simulink model "isubsystem_main"  (R2014b)
settings: Solver=ode45  StartTime=0.0  StopTime=5  FixedStep=0.001  RelTol=1e-3
undefined symbols (not defined in the file): v1, v10, v11, v12, v13, v14, v15, v16, v17, v18, v19, v2, v20, v21, v22, v3, v4, v5, v6, v7, v8, v9
(part 1 of 2)
settings Model: Creator=QiuJiongzhi  LastModifiedBy=QiuJiongzhi
settings SolverCC: ZeroCrossControl=DisableAll

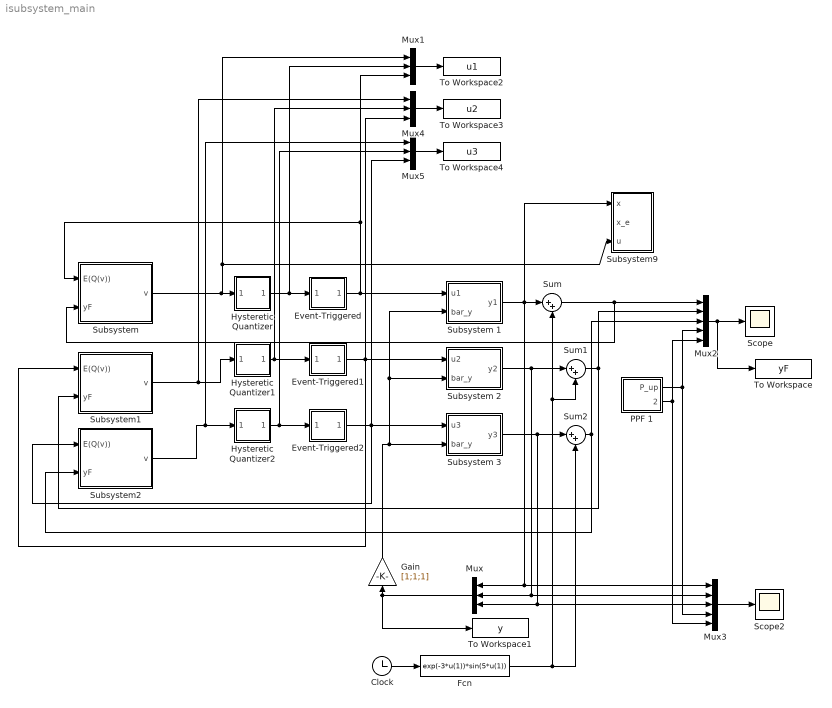
== system isubsystem_main ==
  Clock : Clock
  Event-Triggered : Subsystem
      mask Display: fprintf('E(μ)');
  Event-Triggered1 : Subsystem
      mask Display: fprintf('E(μ)');
  Event-Triggered2 : Subsystem
      mask Display: fprintf('E(μ)');
  Fcn : Fcn  Expr=exp(-3*u(1))*sin(5*u(1))
  Gain : Gain  Gain=[1;1;1]
  Hysteretic Quantizer : Subsystem
      mask Display: fprintf('Q(μ)')
  Hysteretic Quantizer1 : Subsystem
      mask Display: fprintf('Q(μ)')
  Hysteretic Quantizer2 : Subsystem
      mask Display: fprintf('Q(μ)')
  Mux{,1,4..5} (4 alike) : Mux  Inputs=3
  Mux2 : Mux  Inputs=5
  Mux3 : Mux  Inputs=5
  PPF 1 : Subsystem  mask{psi0=1, psiinf=0.05, T=1.5, q=0.1}
  Scope : Scope
      settings: ShowLegends=on  YMin=-1  YMax=1
  Scope2 : Scope
      settings: ShowLegends=on  YMin=-1  YMax=1  SaveName=ScopeData3
  Subsystem : Subsystem
  Subsystem 1 : Subsystem  mask{x1_0=0.5, x2_0=0.3}
      mask prompts: x1_0 "x1(0)"; x2_0 "x2(0)"
  Subsystem 2 : Subsystem  mask{x1_0=0.5, x2_0=0.45}
      mask prompts: x1_0 "x1(0)"; x2_0 "x2(0)"
  Subsystem 3 : Subsystem  mask{x1_0=0.5, x2_0=0.3}
      mask prompts: x1_0 "x1(0)"; x2_0 "x2(0)"
  Subsystem1 : Subsystem
  Subsystem2 : Subsystem
  Subsystem9 : Subsystem
  Sum : Sum  Inputs=|++
  Sum1 : Sum  Inputs=|++
  Sum2 : Sum  Inputs=|++
  To Workspace : ToWorkspace  VariableName=yF  SaveFormat=Structure With Time  SampleTime=-1
  To Workspace1 : ToWorkspace  VariableName=y  SaveFormat=Structure With Time  SampleTime=-1
  To Workspace2 : ToWorkspace  VariableName=u1  SaveFormat=Structure With Time  SampleTime=-1
  To Workspace3 : ToWorkspace  VariableName=u2  SaveFormat=Structure With Time  SampleTime=-1
  To Workspace4 : ToWorkspace  VariableName=u3  SaveFormat=Structure With Time  SampleTime=-1
  wires:
  Sum/1 -> Mux2/1, Subsystem/2(yF)
  Clock/1 -> Fcn/1
  Fcn/1 -> Sum1/2, Sum/2, Sum2/2
  Mux/1 -> To Workspace1/1, Gain/1
  Mux1/1 -> To Workspace2/1
  Hysteretic Quantizer/1(Q(\miu)) -> Mux1/2, Event-Triggered/1(In1)
  Event-Triggered/1(Out1) -> Mux1/3, Subsystem/1(E(Q(v))), Subsystem 1/1(u1)
  Subsystem 2/1(y2) -> Mux/2, Mux3/2, Sum1/1
  Subsystem 3/1(y3) -> Mux3/3, Mux/3, Sum2/1
  Subsystem/1(v) -> Mux1/1, Subsystem9/3(u), Hysteretic Quantizer/1(\miu)
  Event-Triggered1/1(Out1) -> Mux4/3, Subsystem1/1(E(Q(v))), Subsystem 2/1(u2)
  Hysteretic Quantizer1/1(Q(\miu)) -> Event-Triggered1/1(In1), Mux4/2
  Subsystem1/1(v) -> Mux4/1, Hysteretic Quantizer1/1(\miu)
  Sum1/1 -> Subsystem1/2(yF), Mux2/2
  Hysteretic Quantizer2/1(Q(\miu)) -> Mux5/2, Event-Triggered2/1(In1)
  Event-Triggered2/1(Out1) -> Mux5/3, Subsystem2/1(E(Q(v))), Subsystem 3/1(u3)
  Subsystem2/1(v) -> Mux5/1, Hysteretic Quantizer2/1(\miu)
  Sum2/1 -> Subsystem2/2(yF), Mux2/3
  Gain/1 -> Subsystem 3/2(bar_y), Subsystem 2/2(bar_y), Subsystem 1/2(bar_y)
  Mux2/1 -> To Workspace/1, Scope/1
  PPF 1/1(P_up) -> Mux2/4, Mux3/4
  PPF 1/2("P_down ") -> Mux2/5, Mux3/5
  Mux3/1 -> Scope2/1
  Subsystem 1/1(y1) -> Sum/1, Mux3/1, Mux/1, Subsystem9/1(x)
  Mux4/1 -> To Workspace3/1
  Mux5/1 -> To Workspace4/1

== system isubsystem_main/Event-Triggered ==
  In1 : Inport
  MATLAB Function : MATLAB Function  TreatAsAtomicUnit=on
  Mux : Mux  Inputs=2
  Scope : Scope
  To Workspace : ToWorkspace  VariableName=triger1  SaveFormat=Structure With Time  SampleTime=-1
  Unit Delay : UnitDelay  SampleTime=-1
  Out1 : Outport
  wires:
  Unit Delay/1 -> MATLAB Function/2(miu_tk)
  In1/1 -> MATLAB Function/1(miu)
  MATLAB Function/1(E_out) -> Unit Delay/1, Out1/1
  Mux/1 -> Scope/1
  MATLAB Function/2(eta) -> Mux/1
  MATLAB Function/3(triger) -> To Workspace/1, Mux/2

== system isubsystem_main/Event-Triggered1 ==
  In1 : Inport
  MATLAB Function : MATLAB Function  TreatAsAtomicUnit=on
  Mux : Mux  Inputs=2
  Scope : Scope
  To Workspace : ToWorkspace  VariableName=triger2  SaveFormat=Structure With Time  SampleTime=-1
  Unit Delay : UnitDelay  SampleTime=-1
  Out1 : Outport
  wires:
  Unit Delay/1 -> MATLAB Function/2(miu_tk)
  In1/1 -> MATLAB Function/1(miu)
  MATLAB Function/1(E_out) -> Unit Delay/1, Out1/1
  Mux/1 -> Scope/1
  MATLAB Function/2(eta) -> Mux/1
  MATLAB Function/3(triger) -> To Workspace/1, Mux/2

== system isubsystem_main/Event-Triggered2 ==
  In1 : Inport
  MATLAB Function : MATLAB Function  TreatAsAtomicUnit=on
  Mux : Mux  Inputs=2
  Scope : Scope
  To Workspace : ToWorkspace  VariableName=triger3  SaveFormat=Structure With Time  SampleTime=-1
  Unit Delay : UnitDelay  SampleTime=-1
  Out1 : Outport
  wires:
  Unit Delay/1 -> MATLAB Function/2(miu_tk)
  In1/1 -> MATLAB Function/1(miu)
  MATLAB Function/1(E_out) -> Unit Delay/1, Out1/1
  Mux/1 -> Scope/1
  MATLAB Function/2(eta) -> Mux/1
  MATLAB Function/3(triger) -> To Workspace/1, Mux/2

== system isubsystem_main/Hysteretic Quantizer ==
  \miu : Inport
  Derivative : Derivative
  MATLAB Function : MATLAB Function  TreatAsAtomicUnit=on
  Unit Delay : UnitDelay  SampleTime=-1
  Q(\miu) : Outport
  wires:
  Unit Delay/1 -> MATLAB Function/2(Output_t)
  \miu/1 -> Derivative/1, MATLAB Function/1(miu)
  MATLAB Function/1(Q_miu) -> Q(\miu)/1, Unit Delay/1
  Derivative/1 -> MATLAB Function/3(dmiu)

== system isubsystem_main/Hysteretic Quantizer1 ==
  \miu : Inport
  Derivative : Derivative
  MATLAB Function : MATLAB Function  TreatAsAtomicUnit=on
  Unit Delay : UnitDelay  SampleTime=-1
  Q(\miu) : Outport
  wires:
  Unit Delay/1 -> MATLAB Function/2(Output_t)
  \miu/1 -> Derivative/1, MATLAB Function/1(miu)
  MATLAB Function/1(Q_miu) -> Q(\miu)/1, Unit Delay/1
  Derivative/1 -> MATLAB Function/3(dmiu)

== system isubsystem_main/Hysteretic Quantizer2 ==
  \miu : Inport
  Derivative : Derivative
  MATLAB Function : MATLAB Function  TreatAsAtomicUnit=on
  Unit Delay : UnitDelay  SampleTime=-1
  Q(\miu) : Outport
  wires:
  Unit Delay/1 -> MATLAB Function/2(Output_t)
  \miu/1 -> Derivative/1, MATLAB Function/1(miu)
  MATLAB Function/1(Q_miu) -> Q(\miu)/1, Unit Delay/1
  Derivative/1 -> MATLAB Function/3(dmiu)

== system isubsystem_main/PPF 1 ==
  Clock1 : Clock
  Constant : Constant  Value=psi0
  Constant1 : Constant  Value=psiinf
  Constant2 : Constant  Value=q
  Constant3 : Constant  Value=T
  MATLAB Function : MATLAB Function  TreatAsAtomicUnit=on
  Saturation : Saturate  UpperLimit=1  LowerLimit=-1
  Saturation1 : Saturate  UpperLimit=1  LowerLimit=-1
  P_up : Outport
  "P_down " : Outport  Port=2
  wires:
  MATLAB Function/1(P_up) -> Saturation/1
  MATLAB Function/2(P_down) -> Saturation1/1
  Clock1/1 -> MATLAB Function/5(t)
  Constant2/1 -> MATLAB Function/4(q)
  Constant1/1 -> MATLAB Function/2(psiinf)
  Constant/1 -> MATLAB Function/1(psi0)
  Constant3/1 -> MATLAB Function/3(T)
  Saturation/1 -> P_up/1
  Saturation1/1 -> "P_down "/1

== system isubsystem_main/Subsystem ==
  E(Q(v)) : Inport
  yF : Inport  Port=2
  Controller1 : Subsystem  mask{k2=v1, b_low=1, b_high=1, li=1, sigma=v2, gamma1=v3, epsilon10=v4, epsilon11=v5, epsilon12=v6, epsilon13=v7, epsilon14=v8, epsilon15=v9, eta0=v10, gamma2=v11, epsilon20=v12, epsilon22=v13, epsilon23=v14, epsilon24=v15, epsilon25=v16, l1=0.2, l2=1.5, w=v17}
      mask DialogControl Container3 Prompt: α_1
      mask DialogControl Container3_copy Prompt: α_n
      mask DialogControl Container4 Prompt: Q(v)
  Fuzzy : Subsystem  mask{Psi=1, eta1=v22}
  "PPF " : Subsystem  mask{psi0=1, psiinf=0.05, T=1.5, q=0.1}
  reduced-order dynamic gain observer : Subsystem  mask{k2=v1, sigma=v2, theta=v18, K=v19, P=1, lP=1, epsilon1=v20, epsilon2=v21, epsilon10=v4, epsilon20=v12, vartheta=0.05}
  v : Outport
  wires:
  Fuzzy/2(Xi) -> Controller1/8(Xi)
  Fuzzy/1(dW) -> Controller1/7(dW)
  reduced-order dynamic gain observer/2(lambda2) -> Controller1/6(lambda2)
  reduced-order dynamic gain observer/1(dL) -> Controller1/5(dL)
  "PPF "/2("dpsi ") -> Controller1/3(dpsi)
  Controller1/1(v) -> v/1
  "PPF "/1(psi) -> Controller1/2(psi)
  "PPF "/3(ddpsi) -> Controller1/4(ddpsi)
  Controller1/2(z1) -> Fuzzy/2(z1)
  E(Q(v))/1 -> reduced-order dynamic gain observer/1(u)
  yF/1 -> Fuzzy/1(yF), Controller1/1(yF), reduced-order dynamic gain observer/2(yF)

== system isubsystem_main/Subsystem 1 ==
  u1 : Inport
  bar_y : Inport  Port=2
  Integrator : Integrator  InitialCondition=x1_0
  Integrator1 : Integrator  InitialCondition=x2_0
  MATLAB Function : MATLAB Function  TreatAsAtomicUnit=on
  To Workspace : ToWorkspace  VariableName=x21  SaveFormat=Structure With Time  SampleTime=-1
  y1 : Outport
  wires:
  Integrator1/1 -> To Workspace/1, MATLAB Function/2(x2)
  MATLAB Function/2(dx2) -> Integrator1/1
  Integrator/1 -> MATLAB Function/1(x1)
  MATLAB Function/1(dx1) -> Integrator/1
  MATLAB Function/3(y) -> y1/1
  u1/1 -> MATLAB Function/3(u)
  bar_y/1 -> MATLAB Function/4(bar_y)

== system isubsystem_main/Subsystem 2 ==
  u2 : Inport
  bar_y : Inport  Port=2
  Integrator : Integrator  InitialCondition=x1_0
  Integrator1 : Integrator  InitialCondition=x2_0
  MATLAB Function : MATLAB Function  TreatAsAtomicUnit=on
  To Workspace : ToWorkspace  VariableName=x22  SaveFormat=Structure With Time  SampleTime=-1
  y2 : Outport
  wires:
  Integrator1/1 -> To Workspace/1, MATLAB Function/2(x2)
  MATLAB Function/2(dx2) -> Integrator1/1
  Integrator/1 -> MATLAB Function/1(x1)
  MATLAB Function/1(dx1) -> Integrator/1
  MATLAB Function/3(y) -> y2/1
  u2/1 -> MATLAB Function/3(u)
  bar_y/1 -> MATLAB Function/4(bar_y)

== system isubsystem_main/Subsystem 3 ==
  u3 : Inport
  bar_y : Inport  Port=2
  Integrator : Integrator  InitialCondition=x1_0
  Integrator1 : Integrator  InitialCondition=x2_0
  MATLAB Function : MATLAB Function  TreatAsAtomicUnit=on
  To Workspace : ToWorkspace  VariableName=x23  SaveFormat=Structure With Time  SampleTime=-1
  y3 : Outport
  wires:
  Integrator1/1 -> MATLAB Function/2(x2), To Workspace/1
  MATLAB Function/2(dx2) -> Integrator1/1
  Integrator/1 -> MATLAB Function/1(x1)
  MATLAB Function/1(dx1) -> Integrator/1
  MATLAB Function/3(y) -> y3/1
  u3/1 -> MATLAB Function/3(u)
  bar_y/1 -> MATLAB Function/4(bar_y)

== system isubsystem_main/Subsystem1 ==
  E(Q(v)) : Inport
  yF : Inport  Port=2
  Controller1 : Subsystem  mask{k2=v1, b_low=1, b_high=1, li=1, sigma=v2, gamma1=v3, epsilon10=v4, epsilon11=v5, epsilon12=v6, epsilon13=v7, epsilon14=v8, epsilon15=v9, eta0=v10, gamma2=v11, epsilon20=v12, epsilon22=v13, epsilon23=v14, epsilon24=v15, epsilon25=v16, l1=0.2, l2=1.5, w=v17}
      mask DialogControl Container3 Prompt: α_1
      mask DialogControl Container3_copy Prompt: α_n
      mask DialogControl Container4 Prompt: Q(v)
  Fuzzy : Subsystem  mask{Psi=1, eta1=v22}
  "PPF " : Subsystem  mask{psi0=1, psiinf=0.05, T=1.5, q=0.1}
  reduced-order dynamic gain observer : Subsystem  mask{k2=v1, sigma=v2, theta=v18, K=v19, P=1, lP=1, epsilon1=v20, epsilon2=v21, epsilon10=v4, epsilon20=v12, vartheta=0.05}
  v : Outport
  wires:
  Fuzzy/2(Xi) -> Controller1/8(Xi)
  Fuzzy/1(dW) -> Controller1/7(dW)
  reduced-order dynamic gain observer/2(lambda2) -> Controller1/6(lambda2)
  reduced-order dynamic gain observer/1(dL) -> Controller1/5(dL)
  "PPF "/2("dpsi ") -> Controller1/3(dpsi)
  Controller1/1(v) -> v/1
  "PPF "/1(psi) -> Controller1/2(psi)
  "PPF "/3(ddpsi) -> Controller1/4(ddpsi)
  Controller1/2(z1) -> Fuzzy/2(z1)
  E(Q(v))/1 -> reduced-order dynamic gain observer/1(u)
  yF/1 -> Fuzzy/1(yF), Controller1/1(yF), reduced-order dynamic gain observer/2(yF)

== system isubsystem_main/Subsystem2 ==
  E(Q(v)) : Inport
  yF : Inport  Port=2
  Controller1 : Subsystem  mask{k2=v1, b_low=1, b_high=1, li=1, sigma=v2, gamma1=v3, epsilon10=v4, epsilon11=v5, epsilon12=v6, epsilon13=v7, epsilon14=v8, epsilon15=v9, eta0=v10, gamma2=v11, epsilon20=v12, epsilon22=v13, epsilon23=v14, epsilon24=v15, epsilon25=v16, l1=0.2, l2=1.5, w=v17}
      mask DialogControl Container3 Prompt: α_1
      mask DialogControl Container3_copy Prompt: α_n
      mask DialogControl Container4 Prompt: Q(v)
  Fuzzy : Subsystem  mask{Psi=1, eta1=v22}
  "PPF " : Subsystem  mask{psi0=1, psiinf=0.05, T=1.5, q=0.1}
  reduced-order dynamic gain observer : Subsystem  mask{k2=v1, sigma=v2, theta=v18, K=v19, P=1, lP=1, epsilon1=v20, epsilon2=v21, epsilon10=v4, epsilon20=v12, vartheta=0.05}
  v : Outport
  wires:
  Fuzzy/2(Xi) -> Controller1/8(Xi)
  Fuzzy/1(dW) -> Controller1/7(dW)
  reduced-order dynamic gain observer/2(lambda2) -> Controller1/6(lambda2)
  reduced-order dynamic gain observer/1(dL) -> Controller1/5(dL)
  "PPF "/2("dpsi ") -> Controller1/3(dpsi)
  Controller1/1(v) -> v/1
  "PPF "/1(psi) -> Controller1/2(psi)
  "PPF "/3(ddpsi) -> Controller1/4(ddpsi)
  Controller1/2(z1) -> Fuzzy/2(z1)
  E(Q(v))/1 -> reduced-order dynamic gain observer/1(u)
  yF/1 -> Fuzzy/1(yF), Controller1/1(yF), reduced-order dynamic gain observer/2(yF)

== system isubsystem_main/Subsystem9 ==
  x : Inport
  x_e : Inport  Port=2
  u : Inport  Port=3
  Abs1 : Abs
  Abs3 : Abs
  Clock : Clock
  Gain2 : Gain  Gain=2
  Integrator1 : Integrator
  Integrator5 : Integrator
  Product1 : Product
  Product3 : Product
  Sum : Sum  Inputs=|+-
  Sum of Elements : Sum  Inputs=+
  Sum of Elements1 : Sum  Inputs=+
  Sum1 : Sum  Inputs=|++
  To Workspace : ToWorkspace  VariableName=simout1  SaveFormat=Structure With Time  SampleTime=-1
  f2 : Scope
      settings: TimeRange=24.44047636723186  YMin=-2  YMax=3  SaveName=f2
  wires:
  Clock/1 -> Product1/1, Product3/1
  Abs3/1 -> Integrator5/1
  x/1 -> Sum/1
  x_e/1 -> Sum/2
  Sum/1 -> Product3/2
  Sum1/1 -> To Workspace/1, f2/1
  u/1 -> Product1/2
  Product1/1 -> Abs1/1
  Abs1/1 -> Integrator1/1
  Integrator1/1 -> Sum of Elements1/1
  Sum of Elements/1 -> Sum1/1
  Sum of Elements1/1 -> Gain2/1
  Gain2/1 -> Sum1/2
  Integrator5/1 -> Sum of Elements/1
  Product3/1 -> Abs3/1

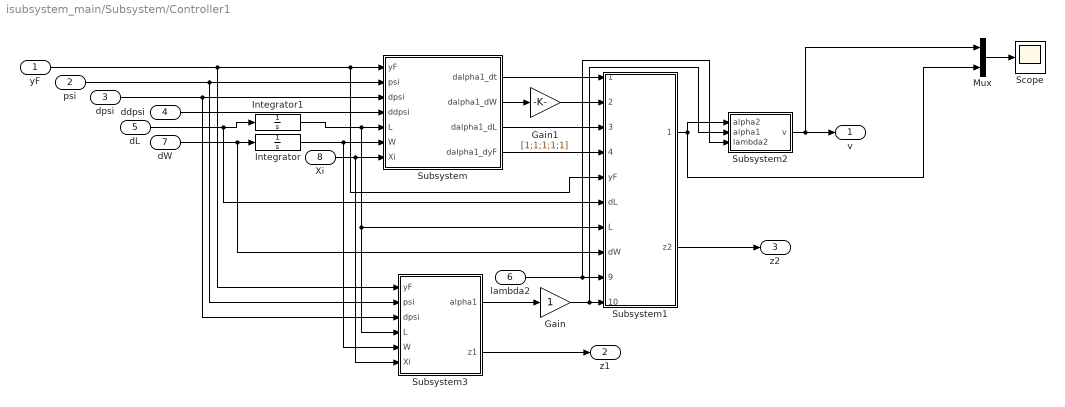
== system isubsystem_main/Subsystem/Controller1 ==
  yF : Inport
  psi : Inport  Port=2
  dpsi : Inport  Port=3
  ddpsi : Inport  Port=4
  dL : Inport  Port=5
  lambda2 : Inport  Port=6
  dW : Inport  Port=7
  Xi : Inport  Port=8
  Gain : Gain
  Gain1 : Gain  Gain=[1;1;1;1;1]
  Integrator : Integrator  InitialCondition=[0;0;0;0;0]
  Integrator1 : Integrator  InitialCondition=1
  Mux : Mux  Inputs=2
  Scope : Scope
      settings: YMin=-1500  YMax=500
  Subsystem : Subsystem
  Subsystem1 : Subsystem
  Subsystem2 : Subsystem
  Subsystem3 : Subsystem
  v : Outport
  z1 : Outport  Port=2
  z2 : Outport  Port=3
  wires:
  yF/1 -> Subsystem3/1(yF), Subsystem1/5(yF), Subsystem/1(yF)
  psi/1 -> Subsystem3/2(psi), Subsystem/2(psi)
  dpsi/1 -> Subsystem3/3(dpsi), Subsystem/3(dpsi)
  dL/1 -> Subsystem1/6(dL), Integrator1/1
  Xi/1 -> Subsystem3/6(Xi), Subsystem/7(Xi)
  Integrator/1 -> Subsystem3/5(W), Subsystem/6(W)
  Integrator1/1 -> Subsystem3/4(L), Subsystem1/7(L), Subsystem/5(L)
  dW/1 -> Subsystem1/8(dW), Integrator/1
  Subsystem/1(dalpha1_dt) -> Subsystem1/1(dalpha1_dt)
  Subsystem/2(dalpha1_dW) -> Gain1/1
  Subsystem/3(dalpha1_dL) -> Subsystem1/3(dalpha1_dL)
  Subsystem/4(dalpha1_dyF) -> Subsystem1/4(dalpha1_dyF)
  lambda2/1 -> Subsystem2/3(lambda2), Subsystem1/9(lambda2)
  Subsystem3/1(alpha1) -> Gain/1
  Subsystem1/1(alpha2) -> Subsystem2/1(alpha2), Mux/2
  Subsystem1/2(z2) -> z2/1
  Subsystem3/2(z1) -> z1/1
  ddpsi/1 -> Subsystem/4(ddpsi)
  Gain/1 -> Subsystem2/2(alpha1), Subsystem1/10(alpha1)
  Gain1/1 -> Subsystem1/2(dalpha1_dW)
  Subsystem2/1(v) -> Mux/1, v/1
  Mux/1 -> Scope/1

== system isubsystem_main/Subsystem/Fuzzy ==
  yF : Inport
  z1 : Inport  Port=2
  Constant1 : Constant  Value=Psi
  Constant3 : Constant  Value=eta1
  Gain : Gain  Gain=[1;1;1;1;1]
  Gain1 : Gain  Gain=[1;1;1;1;1]
  Integrator : Integrator  InitialCondition=[0;0;0;0;0]
  MATLAB Function : MATLAB Function  TreatAsAtomicUnit=on
  To Workspace : ToWorkspace  VariableName=W1  SaveFormat=Structure With Time  SampleTime=-1
  dW : Outport
  Xi : Outport  Port=2
  wires:
  MATLAB Function/2(dW) -> Gain1/1, Integrator/1
  yF/1 -> MATLAB Function/2(yF)
  MATLAB Function/1(Xi) -> Gain/1
  Constant1/1 -> MATLAB Function/4(Psi)
  Integrator/1 -> To Workspace/1, MATLAB Function/1(W)
  Constant3/1 -> MATLAB Function/5(eta1)
  z1/1 -> MATLAB Function/3(z1)
  Gain/1 -> Xi/1
  Gain1/1 -> dW/1

== system isubsystem_main/Subsystem/PPF  ==
  Clock1 : Clock
  Constant : Constant  Value=psi0
  Constant1 : Constant  Value=psiinf
  Constant2 : Constant  Value=q
  Constant3 : Constant  Value=T
  MATLAB Function : MATLAB Function  TreatAsAtomicUnit=on
  psi : Outport
  "dpsi " : Outport  Port=2
  ddpsi : Outport  Port=3
  wires:
  MATLAB Function/1(psi) -> psi/1
  MATLAB Function/2(dpsi) -> "dpsi "/1
  Clock1/1 -> MATLAB Function/5(t)
  Constant2/1 -> MATLAB Function/4(q)
  Constant1/1 -> MATLAB Function/2(psiinf)
  Constant/1 -> MATLAB Function/1(psi0)
  MATLAB Function/3(ddpsi) -> ddpsi/1
  Constant3/1 -> MATLAB Function/3(T)

== system isubsystem_main/Subsystem/reduced-order dynamic gain observer ==
  u : Inport
  yF : Inport  Port=2
  Constant : Constant  Value=k2
  Integrator : Integrator
  MATLAB Function : MATLAB Function  TreatAsAtomicUnit=on
  Mux : Mux  Inputs=2
  Subsystem : Subsystem
  To Workspace : ToWorkspace  VariableName=x2_e1  SaveFormat=Structure With Time  SampleTime=-1
  To Workspace1 : ToWorkspace  VariableName=L1  SaveFormat=Structure With Time  SampleTime=-1
  dL : Outport
  lambda2 : Outport  Port=2
  wires:
  yF/1 -> Subsystem/1(yF), MATLAB Function/3(yF)
  u/1 -> MATLAB Function/2(u)
  Subsystem/1(L) -> To Workspace1/1, MATLAB Function/5(L)
  Constant/1 -> MATLAB Function/4(k2)
  Integrator/1 -> Mux/2, lambda2/1, MATLAB Function/1(lambda2)
  MATLAB Function/1(dlambda2) -> Integrator/1
  Subsystem/2(dL) -> dL/1, MATLAB Function/6(dL)
  Mux/1 -> To Workspace/1
  MATLAB Function/2(x2_e) -> Mux/1

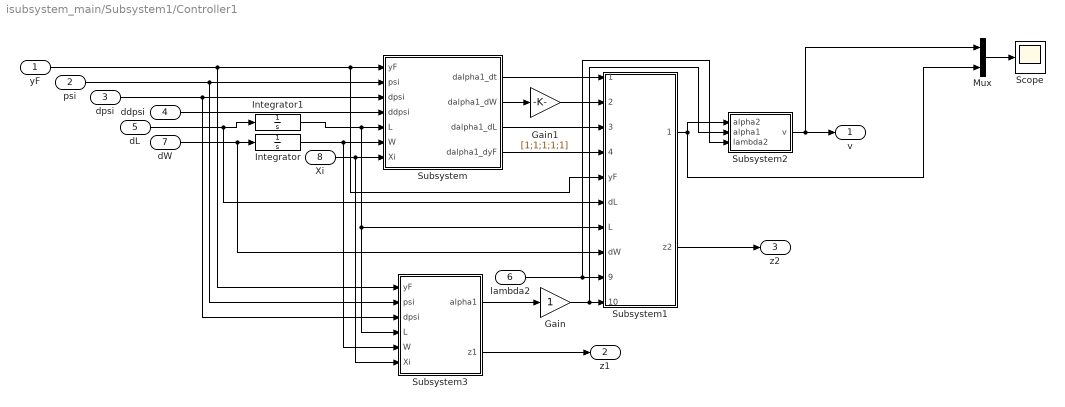
== system isubsystem_main/Subsystem1/Controller1 ==
  yF : Inport
  psi : Inport  Port=2
  dpsi : Inport  Port=3
  ddpsi : Inport  Port=4
  dL : Inport  Port=5
  lambda2 : Inport  Port=6
  dW : Inport  Port=7
  Xi : Inport  Port=8
  Gain : Gain
  Gain1 : Gain  Gain=[1;1;1;1;1]
  Integrator : Integrator  InitialCondition=[0;0;0;0;0]
  Integrator1 : Integrator  InitialCondition=1
  Mux : Mux  Inputs=2
  Scope : Scope
      settings: YMin=-1500  YMax=500
  Subsystem : Subsystem
  Subsystem1 : Subsystem
  Subsystem2 : Subsystem
  Subsystem3 : Subsystem
  v : Outport
  z1 : Outport  Port=2
  z2 : Outport  Port=3
  wires:
  yF/1 -> Subsystem3/1(yF), Subsystem1/5(yF), Subsystem/1(yF)
  psi/1 -> Subsystem3/2(psi), Subsystem/2(psi)
  dpsi/1 -> Subsystem3/3(dpsi), Subsystem/3(dpsi)
  dL/1 -> Subsystem1/6(dL), Integrator1/1
  Xi/1 -> Subsystem3/6(Xi), Subsystem/7(Xi)
  Integrator/1 -> Subsystem3/5(W), Subsystem/6(W)
  Integrator1/1 -> Subsystem3/4(L), Subsystem1/7(L), Subsystem/5(L)
  dW/1 -> Subsystem1/8(dW), Integrator/1
  Subsystem/1(dalpha1_dt) -> Subsystem1/1(dalpha1_dt)
  Subsystem/2(dalpha1_dW) -> Gain1/1
  Subsystem/3(dalpha1_dL) -> Subsystem1/3(dalpha1_dL)
  Subsystem/4(dalpha1_dyF) -> Subsystem1/4(dalpha1_dyF)
  lambda2/1 -> Subsystem2/3(lambda2), Subsystem1/9(lambda2)
  Subsystem3/1(alpha1) -> Gain/1
  Subsystem1/1(alpha2) -> Subsystem2/1(alpha2), Mux/2
  Subsystem1/2(z2) -> z2/1
  Subsystem3/2(z1) -> z1/1
  ddpsi/1 -> Subsystem/4(ddpsi)
  Gain/1 -> Subsystem2/2(alpha1), Subsystem1/10(alpha1)
  Gain1/1 -> Subsystem1/2(dalpha1_dW)
  Subsystem2/1(v) -> Mux/1, v/1
  Mux/1 -> Scope/1

== system isubsystem_main/Subsystem1/Fuzzy ==
  yF : Inport
  z1 : Inport  Port=2
  Constant1 : Constant  Value=Psi
  Constant3 : Constant  Value=eta1
  Gain : Gain  Gain=[1;1;1;1;1]
  Gain1 : Gain  Gain=[1;1;1;1;1]
  Integrator : Integrator  InitialCondition=[0;0;0;0;0]
  MATLAB Function : MATLAB Function  TreatAsAtomicUnit=on
  To Workspace : ToWorkspace  VariableName=W2  SaveFormat=Structure With Time  SampleTime=-1
  dW : Outport
  Xi : Outport  Port=2
  wires:
  MATLAB Function/2(dW) -> Gain1/1, Integrator/1
  yF/1 -> MATLAB Function/2(yF)
  MATLAB Function/1(Xi) -> Gain/1
  Constant1/1 -> MATLAB Function/4(Psi)
  Integrator/1 -> To Workspace/1, MATLAB Function/1(W)
  Constant3/1 -> MATLAB Function/5(eta1)
  z1/1 -> MATLAB Function/3(z1)
  Gain/1 -> Xi/1
  Gain1/1 -> dW/1

== system isubsystem_main/Subsystem1/PPF  ==
  Clock1 : Clock
  Constant : Constant  Value=psi0
  Constant1 : Constant  Value=psiinf
  Constant2 : Constant  Value=q
  Constant3 : Constant  Value=T
  MATLAB Function : MATLAB Function  TreatAsAtomicUnit=on
  psi : Outport
  "dpsi " : Outport  Port=2
  ddpsi : Outport  Port=3
  wires:
  MATLAB Function/1(psi) -> psi/1
  MATLAB Function/2(dpsi) -> "dpsi "/1
  Clock1/1 -> MATLAB Function/5(t)
  Constant2/1 -> MATLAB Function/4(q)
  Constant1/1 -> MATLAB Function/2(psiinf)
  Constant/1 -> MATLAB Function/1(psi0)
  MATLAB Function/3(ddpsi) -> ddpsi/1
  Constant3/1 -> MATLAB Function/3(T)

== system isubsystem_main/Subsystem1/reduced-order dynamic gain observer ==
  u : Inport
  yF : Inport  Port=2
  Constant : Constant  Value=k2
  Integrator : Integrator
  MATLAB Function : MATLAB Function  TreatAsAtomicUnit=on
  Mux : Mux  Inputs=2
  Subsystem : Subsystem
  To Workspace : ToWorkspace  VariableName=x2_e2  SaveFormat=Structure With Time  SampleTime=-1
  To Workspace1 : ToWorkspace  VariableName=L2  SaveFormat=Structure With Time  SampleTime=-1
  dL : Outport
  lambda2 : Outport  Port=2
  wires:
  yF/1 -> Subsystem/1(yF), MATLAB Function/3(yF)
  u/1 -> MATLAB Function/2(u)
  Constant/1 -> MATLAB Function/4(k2)
  Integrator/1 -> Mux/2, lambda2/1, MATLAB Function/1(lambda2)
  MATLAB Function/1(dlambda2) -> Integrator/1
  Subsystem/2(dL) -> dL/1, MATLAB Function/6(dL)
  Subsystem/1(L) -> To Workspace1/1, MATLAB Function/5(L)
  Mux/1 -> To Workspace/1
  MATLAB Function/2(x2_e) -> Mux/1

== system isubsystem_main/Subsystem2/Controller1 ==
  yF : Inport
  psi : Inport  Port=2
  dpsi : Inport  Port=3
  ddpsi : Inport  Port=4
  dL : Inport  Port=5
  lambda2 : Inport  Port=6
  dW : Inport  Port=7
  Xi : Inport  Port=8
  Gain : Gain
  Gain1 : Gain  Gain=[1;1;1;1;1]
  Integrator : Integrator  InitialCondition=[0;0;0;0;0]
  Integrator1 : Integrator  InitialCondition=1
  Mux : Mux  Inputs=2
  Scope : Scope
      settings: YMin=-1500  YMax=500
  Subsystem : Subsystem
  Subsystem1 : Subsystem
  Subsystem2 : Subsystem
  Subsystem3 : Subsystem
  v : Outport
  z1 : Outport  Port=2
  z2 : Outport  Port=3
  wires:
  yF/1 -> Subsystem3/1(yF), Subsystem1/5(yF), Subsystem/1(yF)
  psi/1 -> Subsystem3/2(psi), Subsystem/2(psi)
  dpsi/1 -> Subsystem3/3(dpsi), Subsystem/3(dpsi)
  dL/1 -> Subsystem1/6(dL), Integrator1/1
  Xi/1 -> Subsystem3/6(Xi), Subsystem/7(Xi)
  Integrator/1 -> Subsystem3/5(W), Subsystem/6(W)
  Integrator1/1 -> Subsystem3/4(L), Subsystem1/7(L), Subsystem/5(L)
  dW/1 -> Subsystem1/8(dW), Integrator/1
  Subsystem/1(dalpha1_dt) -> Subsystem1/1(dalpha1_dt)
  Subsystem/2(dalpha1_dW) -> Gain1/1
  Subsystem/3(dalpha1_dL) -> Subsystem1/3(dalpha1_dL)
  Subsystem/4(dalpha1_dyF) -> Subsystem1/4(dalpha1_dyF)
  lambda2/1 -> Subsystem2/3(lambda2), Subsystem1/9(lambda2)
  Subsystem3/1(alpha1) -> Gain/1
  Subsystem1/1(alpha2) -> Subsystem2/1(alpha2), Mux/2
  Subsystem1/2(z2) -> z2/1
  Subsystem3/2(z1) -> z1/1
  ddpsi/1 -> Subsystem/4(ddpsi)
  Gain/1 -> Subsystem2/2(alpha1), Subsystem1/10(alpha1)
  Gain1/1 -> Subsystem1/2(dalpha1_dW)
  Subsystem2/1(v) -> Mux/1, v/1
  Mux/1 -> Scope/1

== system isubsystem_main/Subsystem2/Fuzzy ==
  yF : Inport
  z1 : Inport  Port=2
  Constant1 : Constant  Value=Psi
  Constant3 : Constant  Value=eta1
  Gain : Gain  Gain=[1;1;1;1;1]
  Gain1 : Gain  Gain=[1;1;1;1;1]
  Integrator : Integrator  InitialCondition=[0;0;0;0;0]
  MATLAB Function : MATLAB Function  TreatAsAtomicUnit=on
  To Workspace : ToWorkspace  VariableName=W3  SaveFormat=Structure With Time  SampleTime=-1
  dW : Outport
  Xi : Outport  Port=2
  wires:
  MATLAB Function/2(dW) -> Gain1/1, Integrator/1
  yF/1 -> MATLAB Function/2(yF)
  MATLAB Function/1(Xi) -> Gain/1
  Constant1/1 -> MATLAB Function/4(Psi)
  Integrator/1 -> MATLAB Function/1(W), To Workspace/1
  Constant3/1 -> MATLAB Function/5(eta1)
  z1/1 -> MATLAB Function/3(z1)
  Gain/1 -> Xi/1
  Gain1/1 -> dW/1

== system isubsystem_main/Subsystem2/PPF  ==
  Clock1 : Clock
  Constant : Constant  Value=psi0
  Constant1 : Constant  Value=psiinf
  Constant2 : Constant  Value=q
  Constant3 : Constant  Value=T
  MATLAB Function : MATLAB Function  TreatAsAtomicUnit=on
  psi : Outport
  "dpsi " : Outport  Port=2
  ddpsi : Outport  Port=3
  wires:
  MATLAB Function/1(psi) -> psi/1
  MATLAB Function/2(dpsi) -> "dpsi "/1
  Clock1/1 -> MATLAB Function/5(t)
  Constant2/1 -> MATLAB Function/4(q)
  Constant1/1 -> MATLAB Function/2(psiinf)
  Constant/1 -> MATLAB Function/1(psi0)
  MATLAB Function/3(ddpsi) -> ddpsi/1
  Constant3/1 -> MATLAB Function/3(T)

== system isubsystem_main/Subsystem2/reduced-order dynamic gain observer ==
  u : Inport
  yF : Inport  Port=2
  Constant : Constant  Value=k2
  Integrator : Integrator
  MATLAB Function : MATLAB Function  TreatAsAtomicUnit=on
  Mux : Mux  Inputs=2
  Subsystem : Subsystem
  To Workspace : ToWorkspace  VariableName=x2_e3  SaveFormat=Structure With Time  SampleTime=-1
  To Workspace1 : ToWorkspace  VariableName=L3  SaveFormat=Structure With Time  SampleTime=-1
  dL : Outport
  lambda2 : Outport  Port=2
  wires:
  yF/1 -> Subsystem/1(yF), MATLAB Function/3(yF)
  u/1 -> MATLAB Function/2(u)
  Constant/1 -> MATLAB Function/4(k2)
  Integrator/1 -> Mux/2, lambda2/1, MATLAB Function/1(lambda2)
  MATLAB Function/1(dlambda2) -> Integrator/1
  Subsystem/2(dL) -> dL/1, MATLAB Function/6(dL)
  Subsystem/1(L) -> To Workspace1/1, MATLAB Function/5(L)
  Mux/1 -> To Workspace/1
  MATLAB Function/2(x2_e) -> Mux/1

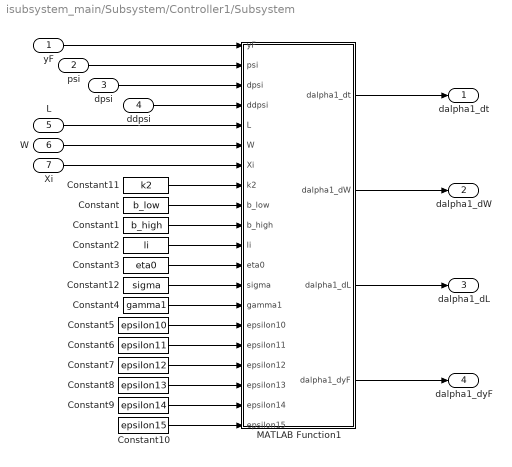
== system isubsystem_main/Subsystem/Controller1/Subsystem ==
  yF : Inport
  psi : Inport  Port=2
  dpsi : Inport  Port=3
  ddpsi : Inport  Port=4
  L : Inport  Port=5
  W : Inport  Port=6
  Xi : Inport  Port=7
  Constant : Constant  Value=b_low
  Constant1 : Constant  Value=b_high
  Constant10 : Constant  Value=epsilon15
  Constant11 : Constant  Value=k2
  Constant12 : Constant  Value=sigma
  Constant2 : Constant  Value=li
  Constant3 : Constant  Value=eta0
  Constant4 : Constant  Value=gamma1
  Constant5 : Constant  Value=epsilon10
  Constant6 : Constant  Value=epsilon11
  Constant7 : Constant  Value=epsilon12
  Constant8 : Constant  Value=epsilon13
  Constant9 : Constant  Value=epsilon14
  MATLAB Function1 : MATLAB Function  TreatAsAtomicUnit=on
  dalpha1_dt : Outport
  dalpha1_dW : Outport  Port=2
  dalpha1_dL : Outport  Port=3
  dalpha1_dyF : Outport  Port=4
  wires:
  MATLAB Function1/4(dalpha1_dyF) -> dalpha1_dyF/1
  MATLAB Function1/2(dalpha1_dW) -> dalpha1_dW/1
  MATLAB Function1/3(dalpha1_dL) -> dalpha1_dL/1
  Constant10/1 -> MATLAB Function1/20(epsilon15)
  W/1 -> MATLAB Function1/6(W)
  MATLAB Function1/1(dalpha1_dt) -> dalpha1_dt/1
  yF/1 -> MATLAB Function1/1(yF)
  Constant/1 -> MATLAB Function1/9(b_low)
  Constant9/1 -> MATLAB Function1/19(epsilon14)
  Constant2/1 -> MATLAB Function1/11(li)
  Constant3/1 -> MATLAB Function1/12(eta0)
  Constant1/1 -> MATLAB Function1/10(b_high)
  Constant5/1 -> MATLAB Function1/15(epsilon10)
  Constant8/1 -> MATLAB Function1/18(epsilon13)
  psi/1 -> MATLAB Function1/2(psi)
  Constant6/1 -> MATLAB Function1/16(epsilon11)
  L/1 -> MATLAB Function1/5(L)
  Constant12/1 -> MATLAB Function1/13(sigma)
  Constant4/1 -> MATLAB Function1/14(gamma1)
  Xi/1 -> MATLAB Function1/7(Xi)
  Constant11/1 -> MATLAB Function1/8(k2)
  dpsi/1 -> MATLAB Function1/3(dpsi)
  Constant7/1 -> MATLAB Function1/17(epsilon12)
  ddpsi/1 -> MATLAB Function1/4(ddpsi)

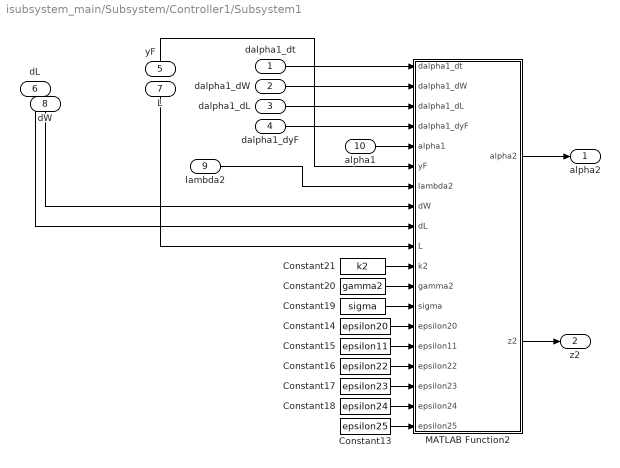
== system isubsystem_main/Subsystem/Controller1/Subsystem1 ==
  dalpha1_dt : Inport
  dalpha1_dW : Inport  Port=2
  dalpha1_dL : Inport  Port=3
  dalpha1_dyF : Inport  Port=4
  yF : Inport  Port=5
  dL : Inport  Port=6
  L : Inport  Port=7
  dW : Inport  Port=8
  lambda2 : Inport  Port=9
  alpha1 : Inport  Port=10
  Constant13 : Constant  Value=epsilon25
  Constant14 : Constant  Value=epsilon20
  Constant15 : Constant  Value=epsilon11
  Constant16 : Constant  Value=epsilon22
  Constant17 : Constant  Value=epsilon23
  Constant18 : Constant  Value=epsilon24
  Constant19 : Constant  Value=sigma
  Constant20 : Constant  Value=gamma2
  Constant21 : Constant  Value=k2
  MATLAB Function2 : MATLAB Function  TreatAsAtomicUnit=on
  alpha2 : Outport
  z2 : Outport  Port=2
  wires:
  Constant19/1 -> MATLAB Function2/13(sigma)
  Constant17/1 -> MATLAB Function2/17(epsilon23)
  Constant13/1 -> MATLAB Function2/19(epsilon25)
  dL/1 -> MATLAB Function2/9(dL)
  MATLAB Function2/1(alpha2) -> alpha2/1
  yF/1 -> MATLAB Function2/6(yF)
  L/1 -> MATLAB Function2/10(L)
  dW/1 -> MATLAB Function2/8(dW)
  dalpha1_dW/1 -> MATLAB Function2/2(dalpha1_dW)
  dalpha1_dyF/1 -> MATLAB Function2/4(dalpha1_dyF)
  dalpha1_dL/1 -> MATLAB Function2/3(dalpha1_dL)
  Constant20/1 -> MATLAB Function2/12(gamma2)
  Constant21/1 -> MATLAB Function2/11(k2)
  Constant18/1 -> MATLAB Function2/18(epsilon24)
  Constant16/1 -> MATLAB Function2/16(epsilon22)
  Constant14/1 -> MATLAB Function2/14(epsilon20)
  Constant15/1 -> MATLAB Function2/15(epsilon11)
  lambda2/1 -> MATLAB Function2/7(lambda2)
  dalpha1_dt/1 -> MATLAB Function2/1(dalpha1_dt)
  alpha1/1 -> MATLAB Function2/5(alpha1)
  MATLAB Function2/2(z2) -> z2/1

== system isubsystem_main/Subsystem/Controller1/Subsystem2 ==
  alpha2 : Inport
  alpha1 : Inport  Port=2
  lambda2 : Inport  Port=3
  Constant : Constant  Value=l1
  Constant1 : Constant  Value=l2
  Constant2 : Constant  Value=w
  MATLAB Function : MATLAB Function  TreatAsAtomicUnit=on
  v : Outport
  wires:
  Constant1/1 -> MATLAB Function/5(l2)
  lambda2/1 -> MATLAB Function/3(lambda2)
  alpha1/1 -> MATLAB Function/2(alpha1)
  Constant/1 -> MATLAB Function/4(l1)
  Constant2/1 -> MATLAB Function/6(w)
  MATLAB Function/1(v) -> v/1
  alpha2/1 -> MATLAB Function/1(alpha2)

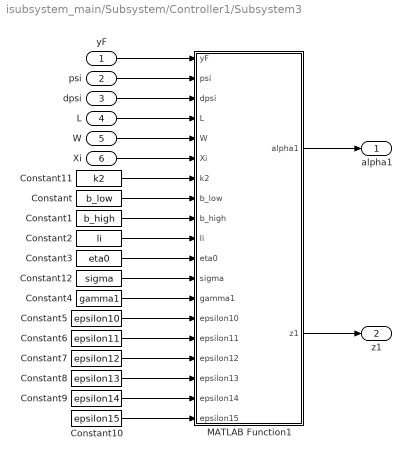
== system isubsystem_main/Subsystem/Controller1/Subsystem3 ==
  yF : Inport
  psi : Inport  Port=2
  dpsi : Inport  Port=3
  L : Inport  Port=4
  W : Inport  Port=5
  Xi : Inport  Port=6
  Constant : Constant  Value=b_low
  Constant1 : Constant  Value=b_high
  Constant10 : Constant  Value=epsilon15
  Constant11 : Constant  Value=k2
  Constant12 : Constant  Value=sigma
  Constant2 : Constant  Value=li
  Constant3 : Constant  Value=eta0
  Constant4 : Constant  Value=gamma1
  Constant5 : Constant  Value=epsilon10
  Constant6 : Constant  Value=epsilon11
  Constant7 : Constant  Value=epsilon12
  Constant8 : Constant  Value=epsilon13
  Constant9 : Constant  Value=epsilon14
  MATLAB Function1 : MATLAB Function  TreatAsAtomicUnit=on
  alpha1 : Outport
  z1 : Outport  Port=2
  wires:
  Constant3/1 -> MATLAB Function1/11(eta0)
  Constant9/1 -> MATLAB Function1/18(epsilon14)
  Constant/1 -> MATLAB Function1/8(b_low)
  Constant1/1 -> MATLAB Function1/9(b_high)
  Constant2/1 -> MATLAB Function1/10(li)
  Constant5/1 -> MATLAB Function1/14(epsilon10)
  Constant11/1 -> MATLAB Function1/7(k2)
  psi/1 -> MATLAB Function1/2(psi)
  L/1 -> MATLAB Function1/4(L)
  Constant10/1 -> MATLAB Function1/19(epsilon15)
  Xi/1 -> MATLAB Function1/6(Xi)
  MATLAB Function1/1(alpha1) -> alpha1/1
  Constant6/1 -> MATLAB Function1/15(epsilon11)
  Constant4/1 -> MATLAB Function1/13(gamma1)
  Constant8/1 -> MATLAB Function1/17(epsilon13)
  W/1 -> MATLAB Function1/5(W)
  dpsi/1 -> MATLAB Function1/3(dpsi)
  Constant7/1 -> MATLAB Function1/16(epsilon12)
  yF/1 -> MATLAB Function1/1(yF)
  Constant12/1 -> MATLAB Function1/12(sigma)
  MATLAB Function1/2(z1) -> z1/1

== system isubsystem_main/Subsystem/reduced-order dynamic gain observer/Subsystem ==
  yF : Inport
  Constant : Constant  Value=norm(P,2)*epsilon1^2/lP + ((2*epsilon10^2)^(-1)+(2*epsilon20^2)^(-1))/lP + norm(P,2)*(epsilon2^4)/(lP*epsilon2^2)
  Constant1 : Constant  Value=sigma
  Constant10 : Constant  Value=vartheta
  Constant2 : Constant  Value=theta
  Constant3 : Constant  Value=K
  Constant4 : Constant  Value=P
  Constant5 : Constant  Value=lP
  Constant6 : Constant  Value=epsilon1
  Constant7 : Constant  Value=epsilon2
  Constant8 : Constant  Value=epsilon10
  Constant9 : Constant  Value=epsilon20
  Display : Display
  Integrator1 : Integrator  InitialCondition=1
  MATLAB Function2 : MATLAB Function  TreatAsAtomicUnit=on
  Saturation : Saturate  UpperLimit=theta+norm(P,2)*epsilon1^2/lP + ((2*epsilon10^2)^(-1)+(2*epsilon20^2)^(-1))/lP + norm(P,2)*(epsilon2^4)/(lP*epsilon2^2)  LowerLimit=theta
  Saturation1 : Saturate  UpperLimit=inf  LowerLimit=0
  Sum : Sum  Inputs=|++
  L : Outport
  dL : Outport  Port=2
  wires:
  Constant5/1 -> MATLAB Function2/7(lP)
  Constant1/1 -> MATLAB Function2/3(sigma)
  Constant10/1 -> MATLAB Function2/12(vartheta)
  Constant2/1 -> Sum/1
  Constant8/1 -> MATLAB Function2/10(epsilon10)
  Constant7/1 -> MATLAB Function2/9(epsilon2)
  Constant4/1 -> MATLAB Function2/6(P)
  Constant3/1 -> Saturation/1
  Integrator1/1 -> L/1, MATLAB Function2/1(L)
  Constant6/1 -> MATLAB Function2/8(epsilon1)
  MATLAB Function2/1(dL) -> Saturation1/1
  Constant9/1 -> MATLAB Function2/11(epsilon20)
  yF/1 -> MATLAB Function2/2(yF)
  Sum/1 -> MATLAB Function2/4(theta)
  Constant/1 -> Display/1, Sum/2
  Saturation/1 -> MATLAB Function2/5(K)
  Saturation1/1 -> Integrator1/1, dL/1

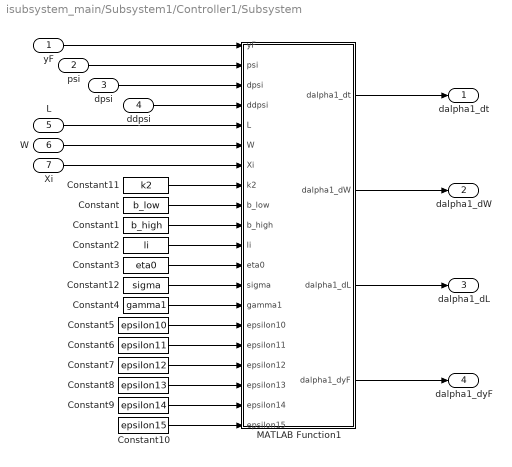
== system isubsystem_main/Subsystem1/Controller1/Subsystem ==
  yF : Inport
  psi : Inport  Port=2
  dpsi : Inport  Port=3
  ddpsi : Inport  Port=4
  L : Inport  Port=5
  W : Inport  Port=6
  Xi : Inport  Port=7
  Constant : Constant  Value=b_low
  Constant1 : Constant  Value=b_high
  Constant10 : Constant  Value=epsilon15
  Constant11 : Constant  Value=k2
  Constant12 : Constant  Value=sigma
  Constant2 : Constant  Value=li
  Constant3 : Constant  Value=eta0
  Constant4 : Constant  Value=gamma1
  Constant5 : Constant  Value=epsilon10
  Constant6 : Constant  Value=epsilon11
  Constant7 : Constant  Value=epsilon12
  Constant8 : Constant  Value=epsilon13
  Constant9 : Constant  Value=epsilon14
  MATLAB Function1 : MATLAB Function  TreatAsAtomicUnit=on
  dalpha1_dt : Outport
  dalpha1_dW : Outport  Port=2
  dalpha1_dL : Outport  Port=3
  dalpha1_dyF : Outport  Port=4
  wires:
  MATLAB Function1/4(dalpha1_dyF) -> dalpha1_dyF/1
  MATLAB Function1/2(dalpha1_dW) -> dalpha1_dW/1
  MATLAB Function1/3(dalpha1_dL) -> dalpha1_dL/1
  Constant10/1 -> MATLAB Function1/20(epsilon15)
  W/1 -> MATLAB Function1/6(W)
  MATLAB Function1/1(dalpha1_dt) -> dalpha1_dt/1
  yF/1 -> MATLAB Function1/1(yF)
  Constant/1 -> MATLAB Function1/9(b_low)
  Constant9/1 -> MATLAB Function1/19(epsilon14)
  Constant2/1 -> MATLAB Function1/11(li)
  Constant3/1 -> MATLAB Function1/12(eta0)
  Constant1/1 -> MATLAB Function1/10(b_high)
  Constant5/1 -> MATLAB Function1/15(epsilon10)
  Constant8/1 -> MATLAB Function1/18(epsilon13)
  psi/1 -> MATLAB Function1/2(psi)
  Constant6/1 -> MATLAB Function1/16(epsilon11)
  L/1 -> MATLAB Function1/5(L)
  Constant12/1 -> MATLAB Function1/13(sigma)
  Constant4/1 -> MATLAB Function1/14(gamma1)
  Xi/1 -> MATLAB Function1/7(Xi)
  Constant11/1 -> MATLAB Function1/8(k2)
  dpsi/1 -> MATLAB Function1/3(dpsi)
  Constant7/1 -> MATLAB Function1/17(epsilon12)
  ddpsi/1 -> MATLAB Function1/4(ddpsi)

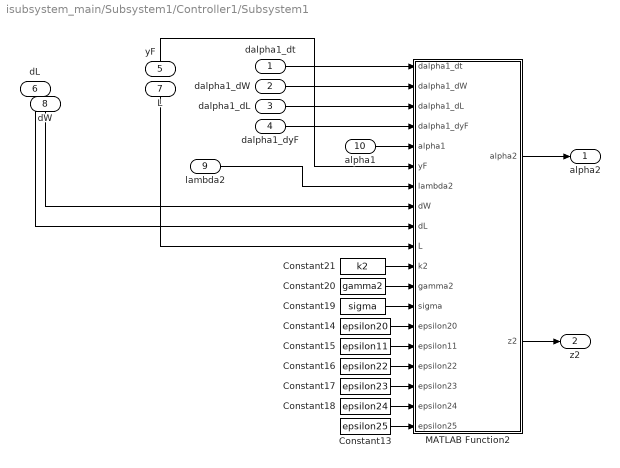
== system isubsystem_main/Subsystem1/Controller1/Subsystem1 ==
  dalpha1_dt : Inport
  dalpha1_dW : Inport  Port=2
  dalpha1_dL : Inport  Port=3
  dalpha1_dyF : Inport  Port=4
  yF : Inport  Port=5
  dL : Inport  Port=6
  L : Inport  Port=7
  dW : Inport  Port=8
  lambda2 : Inport  Port=9
  alpha1 : Inport  Port=10
  Constant13 : Constant  Value=epsilon25
  Constant14 : Constant  Value=epsilon20
  Constant15 : Constant  Value=epsilon11
  Constant16 : Constant  Value=epsilon22
  Constant17 : Constant  Value=epsilon23
  Constant18 : Constant  Value=epsilon24
  Constant19 : Constant  Value=sigma
  Constant20 : Constant  Value=gamma2
  Constant21 : Constant  Value=k2
  MATLAB Function2 : MATLAB Function  TreatAsAtomicUnit=on
  alpha2 : Outport
  z2 : Outport  Port=2
  wires:
  Constant19/1 -> MATLAB Function2/13(sigma)
  Constant17/1 -> MATLAB Function2/17(epsilon23)
  Constant13/1 -> MATLAB Function2/19(epsilon25)
  dL/1 -> MATLAB Function2/9(dL)
  MATLAB Function2/1(alpha2) -> alpha2/1
  yF/1 -> MATLAB Function2/6(yF)
  L/1 -> MATLAB Function2/10(L)
  dW/1 -> MATLAB Function2/8(dW)
  dalpha1_dW/1 -> MATLAB Function2/2(dalpha1_dW)
  dalpha1_dyF/1 -> MATLAB Function2/4(dalpha1_dyF)
  dalpha1_dL/1 -> MATLAB Function2/3(dalpha1_dL)
  Constant20/1 -> MATLAB Function2/12(gamma2)
  Constant21/1 -> MATLAB Function2/11(k2)
  Constant18/1 -> MATLAB Function2/18(epsilon24)
  Constant16/1 -> MATLAB Function2/16(epsilon22)
  Constant14/1 -> MATLAB Function2/14(epsilon20)
  Constant15/1 -> MATLAB Function2/15(epsilon11)
  lambda2/1 -> MATLAB Function2/7(lambda2)
  dalpha1_dt/1 -> MATLAB Function2/1(dalpha1_dt)
  alpha1/1 -> MATLAB Function2/5(alpha1)
  MATLAB Function2/2(z2) -> z2/1

== system isubsystem_main/Subsystem1/Controller1/Subsystem2 ==
  alpha2 : Inport
  alpha1 : Inport  Port=2
  lambda2 : Inport  Port=3
  Constant : Constant  Value=l1
  Constant1 : Constant  Value=l2
  Constant2 : Constant  Value=w
  MATLAB Function : MATLAB Function  TreatAsAtomicUnit=on
  v : Outport
  wires:
  Constant1/1 -> MATLAB Function/5(l2)
  lambda2/1 -> MATLAB Function/3(lambda2)
  alpha1/1 -> MATLAB Function/2(alpha1)
  Constant/1 -> MATLAB Function/4(l1)
  Constant2/1 -> MATLAB Function/6(w)
  MATLAB Function/1(v) -> v/1
  alpha2/1 -> MATLAB Function/1(alpha2)

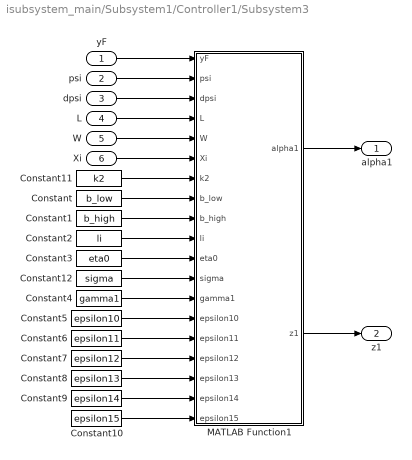
== system isubsystem_main/Subsystem1/Controller1/Subsystem3 ==
  yF : Inport
  psi : Inport  Port=2
  dpsi : Inport  Port=3
  L : Inport  Port=4
  W : Inport  Port=5
  Xi : Inport  Port=6
  Constant : Constant  Value=b_low
  Constant1 : Constant  Value=b_high
  Constant10 : Constant  Value=epsilon15
  Constant11 : Constant  Value=k2
  Constant12 : Constant  Value=sigma
  Constant2 : Constant  Value=li
  Constant3 : Constant  Value=eta0
  Constant4 : Constant  Value=gamma1
  Constant5 : Constant  Value=epsilon10
  Constant6 : Constant  Value=epsilon11
  Constant7 : Constant  Value=epsilon12
  Constant8 : Constant  Value=epsilon13
  Constant9 : Constant  Value=epsilon14
  MATLAB Function1 : MATLAB Function  TreatAsAtomicUnit=on
  alpha1 : Outport
  z1 : Outport  Port=2
  wires:
  Constant3/1 -> MATLAB Function1/11(eta0)
  Constant9/1 -> MATLAB Function1/18(epsilon14)
  Constant/1 -> MATLAB Function1/8(b_low)
  Constant1/1 -> MATLAB Function1/9(b_high)
  Constant2/1 -> MATLAB Function1/10(li)
  Constant5/1 -> MATLAB Function1/14(epsilon10)
  Constant11/1 -> MATLAB Function1/7(k2)
  psi/1 -> MATLAB Function1/2(psi)
  L/1 -> MATLAB Function1/4(L)
  Constant10/1 -> MATLAB Function1/19(epsilon15)
  Xi/1 -> MATLAB Function1/6(Xi)
  MATLAB Function1/1(alpha1) -> alpha1/1
  Constant6/1 -> MATLAB Function1/15(epsilon11)
  Constant4/1 -> MATLAB Function1/13(gamma1)
  Constant8/1 -> MATLAB Function1/17(epsilon13)
  W/1 -> MATLAB Function1/5(W)
  dpsi/1 -> MATLAB Function1/3(dpsi)
  Constant7/1 -> MATLAB Function1/16(epsilon12)
  yF/1 -> MATLAB Function1/1(yF)
  Constant12/1 -> MATLAB Function1/12(sigma)
  MATLAB Function1/2(z1) -> z1/1

== system isubsystem_main/Subsystem1/reduced-order dynamic gain observer/Subsystem ==
  yF : Inport
  Constant : Constant  Value=norm(P,2)*epsilon1^2/lP + ((2*epsilon10^2)^(-1)+(2*epsilon20^2)^(-1))/lP + norm(P,2)*(epsilon2^4)/(lP*epsilon2^2)
  Constant1 : Constant  Value=sigma
  Constant10 : Constant  Value=vartheta
  Constant2 : Constant  Value=theta
  Constant3 : Constant  Value=K
  Constant4 : Constant  Value=P
  Constant5 : Constant  Value=lP
  Constant6 : Constant  Value=epsilon1
  Constant7 : Constant  Value=epsilon2
  Constant8 : Constant  Value=epsilon10
  Constant9 : Constant  Value=epsilon20
  Display : Display
  Integrator1 : Integrator  InitialCondition=1
  MATLAB Function2 : MATLAB Function  TreatAsAtomicUnit=on
  Saturation : Saturate  UpperLimit=theta+norm(P,2)*epsilon1^2/lP + ((2*epsilon10^2)^(-1)+(2*epsilon20^2)^(-1))/lP + norm(P,2)*(epsilon2^4)/(lP*epsilon2^2)  LowerLimit=theta
  Saturation1 : Saturate  UpperLimit=inf  LowerLimit=0
  Sum : Sum  Inputs=|++
  L : Outport
  dL : Outport  Port=2
  wires:
  Constant5/1 -> MATLAB Function2/7(lP)
  Constant1/1 -> MATLAB Function2/3(sigma)
  Constant10/1 -> MATLAB Function2/12(vartheta)
  Constant2/1 -> Sum/1
  Constant8/1 -> MATLAB Function2/10(epsilon10)
  Constant7/1 -> MATLAB Function2/9(epsilon2)
  Constant4/1 -> MATLAB Function2/6(P)
  Constant3/1 -> Saturation/1
  Integrator1/1 -> L/1, MATLAB Function2/1(L)
  Constant6/1 -> MATLAB Function2/8(epsilon1)
  MATLAB Function2/1(dL) -> Saturation1/1
  Constant9/1 -> MATLAB Function2/11(epsilon20)
  yF/1 -> MATLAB Function2/2(yF)
  Sum/1 -> MATLAB Function2/4(theta)
  Constant/1 -> Display/1, Sum/2
  Saturation/1 -> MATLAB Function2/5(K)
  Saturation1/1 -> Integrator1/1, dL/1

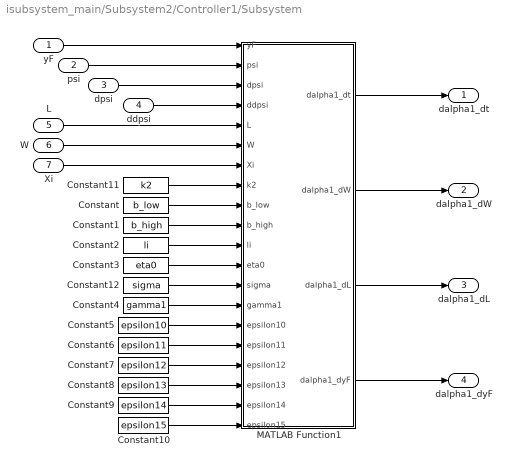
== system isubsystem_main/Subsystem2/Controller1/Subsystem ==
  yF : Inport
  psi : Inport  Port=2
  dpsi : Inport  Port=3
  ddpsi : Inport  Port=4
  L : Inport  Port=5
  W : Inport  Port=6
  Xi : Inport  Port=7
  Constant : Constant  Value=b_low
  Constant1 : Constant  Value=b_high
  Constant10 : Constant  Value=epsilon15
  Constant11 : Constant  Value=k2
  Constant12 : Constant  Value=sigma
  Constant2 : Constant  Value=li
  Constant3 : Constant  Value=eta0
  Constant4 : Constant  Value=gamma1
  Constant5 : Constant  Value=epsilon10
  Constant6 : Constant  Value=epsilon11
  Constant7 : Constant  Value=epsilon12
  Constant8 : Constant  Value=epsilon13
  Constant9 : Constant  Value=epsilon14
  MATLAB Function1 : MATLAB Function  TreatAsAtomicUnit=on
  dalpha1_dt : Outport
  dalpha1_dW : Outport  Port=2
  dalpha1_dL : Outport  Port=3
  dalpha1_dyF : Outport  Port=4
  wires:
  MATLAB Function1/4(dalpha1_dyF) -> dalpha1_dyF/1
  MATLAB Function1/2(dalpha1_dW) -> dalpha1_dW/1
  MATLAB Function1/3(dalpha1_dL) -> dalpha1_dL/1
  Constant10/1 -> MATLAB Function1/20(epsilon15)
  W/1 -> MATLAB Function1/6(W)
  MATLAB Function1/1(dalpha1_dt) -> dalpha1_dt/1
  yF/1 -> MATLAB Function1/1(yF)
  Constant/1 -> MATLAB Function1/9(b_low)
  Constant9/1 -> MATLAB Function1/19(epsilon14)
  Constant2/1 -> MATLAB Function1/11(li)
  Constant3/1 -> MATLAB Function1/12(eta0)
  Constant1/1 -> MATLAB Function1/10(b_high)
  Constant5/1 -> MATLAB Function1/15(epsilon10)
  Constant8/1 -> MATLAB Function1/18(epsilon13)
  psi/1 -> MATLAB Function1/2(psi)
  Constant6/1 -> MATLAB Function1/16(epsilon11)
  L/1 -> MATLAB Function1/5(L)
  Constant12/1 -> MATLAB Function1/13(sigma)
  Constant4/1 -> MATLAB Function1/14(gamma1)
  Xi/1 -> MATLAB Function1/7(Xi)
  Constant11/1 -> MATLAB Function1/8(k2)
  dpsi/1 -> MATLAB Function1/3(dpsi)
  Constant7/1 -> MATLAB Function1/17(epsilon12)
  ddpsi/1 -> MATLAB Function1/4(ddpsi)

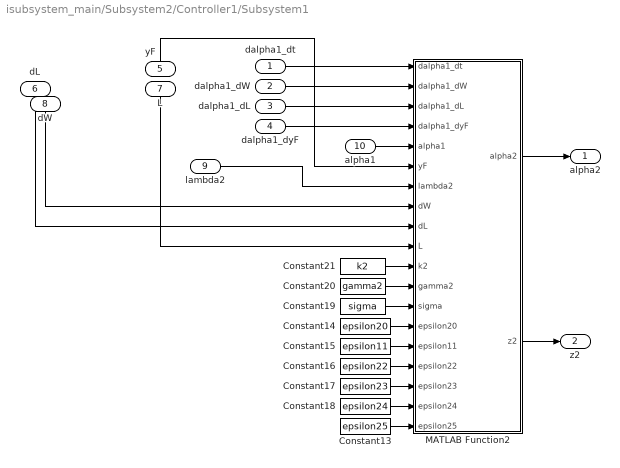
== system isubsystem_main/Subsystem2/Controller1/Subsystem1 ==
  dalpha1_dt : Inport
  dalpha1_dW : Inport  Port=2
  dalpha1_dL : Inport  Port=3
  dalpha1_dyF : Inport  Port=4
  yF : Inport  Port=5
  dL : Inport  Port=6
  L : Inport  Port=7
  dW : Inport  Port=8
  lambda2 : Inport  Port=9
  alpha1 : Inport  Port=10
  Constant13 : Constant  Value=epsilon25
  Constant14 : Constant  Value=epsilon20
  Constant15 : Constant  Value=epsilon11
  Constant16 : Constant  Value=epsilon22
  Constant17 : Constant  Value=epsilon23
  Constant18 : Constant  Value=epsilon24
  Constant19 : Constant  Value=sigma
  Constant20 : Constant  Value=gamma2
  Constant21 : Constant  Value=k2
  MATLAB Function2 : MATLAB Function  TreatAsAtomicUnit=on
  alpha2 : Outport
  z2 : Outport  Port=2
  wires:
  Constant19/1 -> MATLAB Function2/13(sigma)
  Constant17/1 -> MATLAB Function2/17(epsilon23)
  Constant13/1 -> MATLAB Function2/19(epsilon25)
  dL/1 -> MATLAB Function2/9(dL)
  MATLAB Function2/1(alpha2) -> alpha2/1
  yF/1 -> MATLAB Function2/6(yF)
  L/1 -> MATLAB Function2/10(L)
  dW/1 -> MATLAB Function2/8(dW)
  dalpha1_dW/1 -> MATLAB Function2/2(dalpha1_dW)
  dalpha1_dyF/1 -> MATLAB Function2/4(dalpha1_dyF)
  dalpha1_dL/1 -> MATLAB Function2/3(dalpha1_dL)
  Constant20/1 -> MATLAB Function2/12(gamma2)
  Constant21/1 -> MATLAB Function2/11(k2)
  Constant18/1 -> MATLAB Function2/18(epsilon24)
  Constant16/1 -> MATLAB Function2/16(epsilon22)
  Constant14/1 -> MATLAB Function2/14(epsilon20)
  Constant15/1 -> MATLAB Function2/15(epsilon11)
  lambda2/1 -> MATLAB Function2/7(lambda2)
  dalpha1_dt/1 -> MATLAB Function2/1(dalpha1_dt)
  alpha1/1 -> MATLAB Function2/5(alpha1)
  MATLAB Function2/2(z2) -> z2/1

== system isubsystem_main/Subsystem2/Controller1/Subsystem2 ==
  alpha2 : Inport
  alpha1 : Inport  Port=2
  lambda2 : Inport  Port=3
  Constant : Constant  Value=l1
  Constant1 : Constant  Value=l2
  Constant2 : Constant  Value=w
  MATLAB Function : MATLAB Function  TreatAsAtomicUnit=on
  v : Outport
  wires:
  Constant1/1 -> MATLAB Function/5(l2)
  lambda2/1 -> MATLAB Function/3(lambda2)
  alpha1/1 -> MATLAB Function/2(alpha1)
  Constant/1 -> MATLAB Function/4(l1)
  Constant2/1 -> MATLAB Function/6(w)
  MATLAB Function/1(v) -> v/1
  alpha2/1 -> MATLAB Function/1(alpha2)

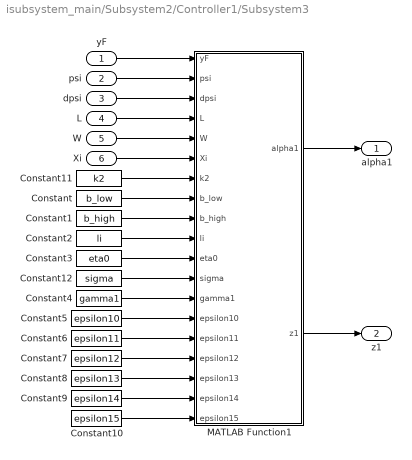
== system isubsystem_main/Subsystem2/Controller1/Subsystem3 ==
  yF : Inport
  psi : Inport  Port=2
  dpsi : Inport  Port=3
  L : Inport  Port=4
  W : Inport  Port=5
  Xi : Inport  Port=6
  Constant : Constant  Value=b_low
  Constant1 : Constant  Value=b_high
  Constant10 : Constant  Value=epsilon15
  Constant11 : Constant  Value=k2
  Constant12 : Constant  Value=sigma
  Constant2 : Constant  Value=li
  Constant3 : Constant  Value=eta0
  Constant4 : Constant  Value=gamma1
  Constant5 : Constant  Value=epsilon10
  Constant6 : Constant  Value=epsilon11
  Constant7 : Constant  Value=epsilon12
  Constant8 : Constant  Value=epsilon13
  Constant9 : Constant  Value=epsilon14
  MATLAB Function1 : MATLAB Function  TreatAsAtomicUnit=on
  alpha1 : Outport
  z1 : Outport  Port=2
  wires:
  Constant3/1 -> MATLAB Function1/11(eta0)
  Constant9/1 -> MATLAB Function1/18(epsilon14)
  Constant/1 -> MATLAB Function1/8(b_low)
  Constant1/1 -> MATLAB Function1/9(b_high)
  Constant2/1 -> MATLAB Function1/10(li)
  Constant5/1 -> MATLAB Function1/14(epsilon10)
  Constant11/1 -> MATLAB Function1/7(k2)
  psi/1 -> MATLAB Function1/2(psi)
  L/1 -> MATLAB Function1/4(L)
  Constant10/1 -> MATLAB Function1/19(epsilon15)
  Xi/1 -> MATLAB Function1/6(Xi)
  MATLAB Function1/1(alpha1) -> alpha1/1
  Constant6/1 -> MATLAB Function1/15(epsilon11)
  Constant4/1 -> MATLAB Function1/13(gamma1)
  Constant8/1 -> MATLAB Function1/17(epsilon13)
  W/1 -> MATLAB Function1/5(W)
  dpsi/1 -> MATLAB Function1/3(dpsi)
  Constant7/1 -> MATLAB Function1/16(epsilon12)
  yF/1 -> MATLAB Function1/1(yF)
  Constant12/1 -> MATLAB Function1/12(sigma)
  MATLAB Function1/2(z1) -> z1/1

== system isubsystem_main/Subsystem2/reduced-order dynamic gain observer/Subsystem ==
  yF : Inport
  Constant : Constant  Value=norm(P,2)*epsilon1^2/lP + ((2*epsilon10^2)^(-1)+(2*epsilon20^2)^(-1))/lP + norm(P,2)*(epsilon2^4)/(lP*epsilon2^2)
  Constant1 : Constant  Value=sigma
  Constant10 : Constant  Value=vartheta
  Constant2 : Constant  Value=theta
  Constant3 : Constant  Value=K
  Constant4 : Constant  Value=P
  Constant5 : Constant  Value=lP
  Constant6 : Constant  Value=epsilon1
  Constant7 : Constant  Value=epsilon2
  Constant8 : Constant  Value=epsilon10
  Constant9 : Constant  Value=epsilon20
  Display : Display
  Integrator1 : Integrator  InitialCondition=1
  MATLAB Function2 : MATLAB Function  TreatAsAtomicUnit=on
  Saturation : Saturate  UpperLimit=theta+norm(P,2)*epsilon1^2/lP + ((2*epsilon10^2)^(-1)+(2*epsilon20^2)^(-1))/lP + norm(P,2)*(epsilon2^4)/(lP*epsilon2^2)  LowerLimit=theta
  Saturation1 : Saturate  UpperLimit=inf  LowerLimit=0
  Sum : Sum  Inputs=|++
  L : Outport
  dL : Outport  Port=2
  wires:
  Constant5/1 -> MATLAB Function2/7(lP)
  Constant1/1 -> MATLAB Function2/3(sigma)
  Constant10/1 -> MATLAB Function2/12(vartheta)
  Constant2/1 -> Sum/1
  Constant8/1 -> MATLAB Function2/10(epsilon10)
  Constant7/1 -> MATLAB Function2/9(epsilon2)
  Constant4/1 -> MATLAB Function2/6(P)
  Constant3/1 -> Saturation/1
  Integrator1/1 -> L/1, MATLAB Function2/1(L)
  Constant6/1 -> MATLAB Function2/8(epsilon1)
  MATLAB Function2/1(dL) -> Saturation1/1
  Constant9/1 -> MATLAB Function2/11(epsilon20)
  yF/1 -> MATLAB Function2/2(yF)
  Sum/1 -> MATLAB Function2/4(theta)
  Constant/1 -> Display/1, Sum/2
  Saturation/1 -> MATLAB Function2/5(K)
  Saturation1/1 -> Integrator1/1, dL/1

== matlab function isubsystem_main/Subsystem 2/MATLAB Function ==
  data: x1 input; x2 input; dx1 output; dx2 output; u input; y output; bar_y input
function [dx1,dx2,y]= fcn(x1,x2,u,bar_y)
%#codegen
y1 = bar_y(1,1);y2 = bar_y(2,1);y3 = bar_y(3,1);
f1 = x1;f2 = x1*x2;
g1 = y2*exp(-y1^2-y3^2);
g2 = y2*y3*sin(y1);
dx1 = x2 + f1 + g1;
dx2 = u + f2 + g2;
y = x1;

== matlab function isubsystem_main/Subsystem 1/MATLAB Function ==
  data: x1 input; x2 input; dx1 output; dx2 output; u input; y output; bar_y input
function [dx1,dx2,y]= fcn(x1,x2,u,bar_y)
%#codegen
y1 = bar_y(1,1);y2 = bar_y(2,1);y3 = bar_y(3,1);
f1 = x1;f2 = x1*x2;
g1 = y1 + y2 + y3;
g2 = y1*cos(y2*y3);
dx1 = x2 + f1 + g1;
dx2 = u + f2 + g2;
y = x1;

== matlab function isubsystem_main/Subsystem 3/MATLAB Function ==
  data: x1 input; x2 input; dx1 output; dx2 output; u input; y output; bar_y input
function [dx1,dx2,y]= fcn(x1,x2,u,bar_y)
%#codegen
y1 = bar_y(1,1);y2 = bar_y(2,1);y3 = bar_y(3,1);
f1 = x1;f2 = x1*x2;
g1 = y3*exp(-y2^2);
g2 = y1*y3;
dx1 = x2 + f1 + g1;
dx2 = u + f2 + g2;
y = x1;
